simulink library "AeroTorqueA"  (R2014b)
settings: Solver=ode45  StartTime=0.0  StopTime=10.0  RelTol=1e-3
libraries: AeroForce_sat x1, LeverArm x1, CrossProd x1
settings Model: Creator=Hp  LastModifiedBy=Hp

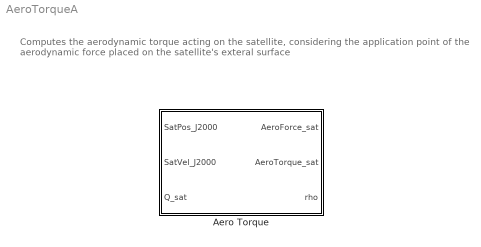
== system AeroTorqueA ==
  note: Computes the aerodynamic torque acting on the satellite,
      | considering the application point of the aerodynamic force
      | placed on the satellite's exteral surface
  Aero Torque : Subsystem

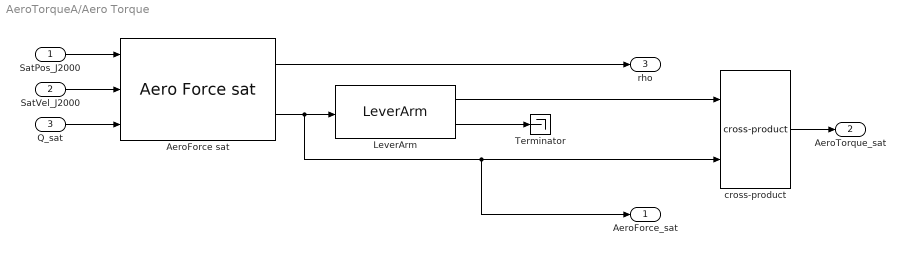
== system AeroTorqueA/Aero Torque ==
  SatPos_J2000 : Inport
  SatVel_J2000 : Inport  Port=2
  Q_sat : Inport  Port=3
  AeroForce sat : AeroForce_sat/Aero Force sat
  LeverArm : LeverArm/LeverArm
  Terminator : Terminator
  cross-product : CrossProd/cross-product
  AeroForce_sat : Outport
  AeroTorque_sat : Outport  Port=2
  rho : Outport  Port=3
  wires:
  SatPos_J2000/1 -> AeroForce sat/1
  AeroForce sat/2 -> AeroForce_sat/1, cross-product/2, LeverArm/1
  Q_sat/1 -> AeroForce sat/3
  SatVel_J2000/1 -> AeroForce sat/2
  LeverArm/1 -> cross-product/1
  AeroForce sat/1 -> rho/1
  cross-product/1 -> AeroTorque_sat/1
  LeverArm/2 -> Terminator/1
